simulink model "model_schuettgut"  (R2020a)
settings: Solver=VariableStepAuto  StartTime=0.0  StopTime=10.0  RelTol=1e-3
libraries: library_schuettgut x4, simulink x2
settings Model: Creator=Jonathan  LastModifiedBy=Jonathan

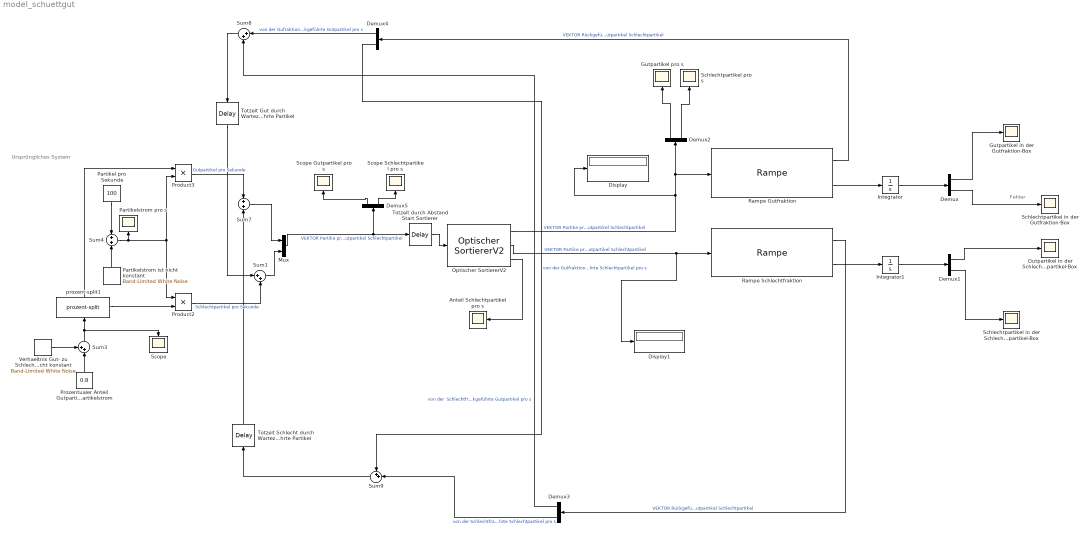
== system model_schuettgut ==
  note: Fehler
  note: Ursprüngliches System
  Anteil Schlechtpartikel pro s : Scope
  Demux{,1..5} (6 alike) : Demux  Outputs=2
  Display : Display
  Display1 : Display
  Gutpartikel in der Gutfraktion-Box : Scope
  Gutpartikel in der Schlechtpartikel-Box : Scope
  Gutpartikel pro s : Scope
  Integrator : Integrator
  Integrator1 : Integrator
  Mux : Mux  Inputs=2
  Optischer SortiererV2 : library_schuettgut/Optischer SortiererV2  SystemSampleTime=-1  Latency=0  AutoFrameSizeCalculation=off
  Partikel pro Sekunde : Constant  Value=100
  Partikelstrom ist nicht konstant : simulink/Sources/Band-Limited White Noise  Cov=[0.2]  Ts=0.1  seed=[23341]
  Partikelstrom pro s : Scope
  Product2 : Product
  Product3 : Product
  Prozentualer Anteil Gutpartikel am gesamten Partikelstrom : Constant  Value=0.8
  Rampe Gutfraktion : library_schuettgut/Rampe  Tag=Rampe  SystemSampleTime=-1  Latency=0  AutoFrameSizeCalculation=off
  Rampe Schlechtfraktion : library_schuettgut/Rampe  Tag=Rampe  SystemSampleTime=-1  Latency=0  AutoFrameSizeCalculation=off
  Schlechtpartikel in der Gutfraktion-Box : Scope
  Schlechtpartikel in der Schlechtpartikel-Box : Scope
  Schlechtpartikel pro s : Scope
  Scope : Scope
  Scope Gutpartikel pro s : Scope
  Scope Schlechtpartikel pro s : Scope
  Sum1 : Sum  Inputs=|++
  Sum3 : Sum  Inputs=++|
  Sum4 : Sum  Inputs=+|+
  Sum7 : Sum  Inputs=+|+
  Sum8 : Sum  Inputs=|++
  Sum9 : Sum  Inputs=++|
  Totzeit durch Abstand Start Sortierer : TransportDelay
  Totzeit Gut durch Wartezeit für zurückgeführte Partikel : TransportDelay
  Totzeit Schlecht durch Wartezeit für zurückgeführte Partikel : TransportDelay
  Verhaeltnis Gut- zu Schlechtpartikel ist nicht konstant : simulink/Sources/Band-Limited White Noise  Cov=[0.0001]  Ts=0.1  seed=[23341]
  prozent-split1 : library_schuettgut/prozent-split  SystemSampleTime=-1  Latency=0  AutoFrameSizeCalculation=off
      settings: PortSchema="{\"entries\":[{\"content\":{\"sides\":[{\"content\":{\"connectorIds\":[\"In1\"]},\"type\":\"ConnectorPlacement.EquallySpacedRectSide\",\"uuid\":\"ab8511c8-9f1d-48ad-bf24-85fd477f0bdd\"},{\"content\":{\"connectorIds\":[\"Out1\"],\"side\":\"RIGHT\"},\"type\":\"ConnectorPlacement.EquallySpacedRectSide\",\"uuid\":\"9ac1a19a-8176-444e-9f4d-7beffa0184e3\"},{\"content\":{\"connectorIds\":[\"Out2\"],\"side\":\"TOP\"},\"type\":\"ConnectorPlacement.EquallySpacedRectSide\",\"uuid\":\"376c2400-f821-4649-ab16-706a2da6117b\"}]},\"type\":\"ConnectorPlacement.EquallySpacedConnector\",\"uuid\":\"f6e72b2d-0467-4732-a018-d51f3a5db703\"}],\"packageUris\":[\"http://schema.mathworks.com/mf0/Connector/19700101\"],\"version\":\"1.0\"}"
  wires:
  Prozentualer Anteil Gutpartikel am gesamten Partikelstrom/1 -> Sum3/2
  Verhaeltnis Gut- zu Schlechtpartikel ist nicht konstant/1 -> Sum3/1
  Sum4/1 -> Product2/1, Product3/2, Partikelstrom pro s/1
  Partikel pro Sekunde/1 -> Sum4/1
  Partikelstrom ist nicht konstant/1 -> Sum4/2
  Product3/1 -> Sum7/1  "Gutpartikel pro Sekunde"
  Totzeit durch Abstand Start Sortierer/1 -> Optischer SortiererV2/1
  Rampe Gutfraktion/1 -> Demux4/1  "VEKTOR Rückgeführte Partikel Gutfraktion pro s Gutpartikel Schlechtpartikel"
  Mux/1 -> Totzeit durch Abstand Start Sortierer/1, Demux5/1  "VEKTOR Partike pro s: Gutpartikel Schlechtpartikel"
  Demux4/1 -> Sum8/1  "von der Gufraktion zurückgeführte Gutpartikel pro s"
  Sum8/1 -> Totzeit Gut durch Wartezeit für zurückgeführte Partikel/1
  Sum9/1 -> Totzeit Schlecht durch Wartezeit für zurückgeführte Partikel/1
  Totzeit Schlecht durch Wartezeit für zurückgeführte Partikel/1 -> Sum7/2
  Rampe Gutfraktion/2 -> Integrator/1
  Optischer SortiererV2/1 -> Display/1, Demux2/1, Rampe Gutfraktion/1  "VEKTOR Partike pro s in der Gutfraktion: Gutpartikel Schlechtpartikel"
  Optischer SortiererV2/2 -> Display1/1, Rampe Schlechtfraktion/1  "VEKTOR Partike pro s in der Schlechtfraktion: Gutpartikel Schlechtpartikel"
  Sum3/1 -> Scope/1, prozent-split1/1
  prozent-split1/1 -> Product3/1
  prozent-split1/2 -> Product2/2
  Product2/1 -> Sum1/2  "Schlechtpartikel pro Sekunde"
  Totzeit Gut durch Wartezeit für zurückgeführte Partikel/1 -> Sum1/1
  Sum1/1 -> Mux/2
  Sum7/1 -> Mux/1
  Demux3/2 -> Sum9/2  "von der Schlechtfraktion zurückgeführte Schlechtpartikel pro s"
  Demux4/2 -> Sum9/1  "von der Gutfraktion zurückgeführte Schlechtpartikel pro s"
  Demux3/1 -> Sum8/2  "von der  Schlechtfraktion zurückgeführte Gutpartikel pro s"
  Demux/1 -> Gutpartikel in der Gutfraktion-Box/1
  Demux/2 -> Schlechtpartikel in der Gutfraktion-Box/1
  Demux1/1 -> Gutpartikel in der Schlechtpartikel-Box/1
  Demux1/2 -> Schlechtpartikel in der Schlechtpartikel-Box/1
  Rampe Schlechtfraktion/2 -> Integrator1/1
  Integrator/1 -> Demux/1
  Integrator1/1 -> Demux1/1
  Demux2/2 -> Schlechtpartikel pro s/1
  Demux2/1 -> Gutpartikel pro s/1
  Rampe Schlechtfraktion/1 -> Demux3/1  "VEKTOR Rückgeführte Partikel Schlechtfraktion pro s Gutpartikel Schlechtpartikel"
  Optischer SortiererV2/3 -> Anteil Schlechtpartikel pro s/1
  Demux5/1 -> Scope Gutpartikel pro s/1
  Demux5/2 -> Scope Schlechtpartikel pro s/1
